simulink model "Controller"  (R2022b)
settings: Solver=FixedStepDiscrete  StartTime=0.0  StopTime=10.0  FixedStep=CONTROL_CONST.dt  RelTol=1e-3
values from neighbouring files (symbols this model uses):
  CONTROL_EXPORT = Simulink.Parameter(CONTROL_EXPORT_VALUE)    [controller_model_init.m]
  CONTROL_PARAM = Simulink.Parameter(CONTROL_PARAM_VALUE)    [controller_model_init.m]
undefined symbols (not defined in the file or in its folder): actuator_cmd, CONTROL_CONST, CONTROL_PARAM_VALUE, ControlMode, DiscIntNeverNeededParam, Discrete, Time, timestamp
libraries: simulink x10, FMT_Model_Lib x2, aerolibasang x1, ctrlSharedLib x1
(part 1 of 2)
settings Model: Creator=19114  LastModifiedBy=19114

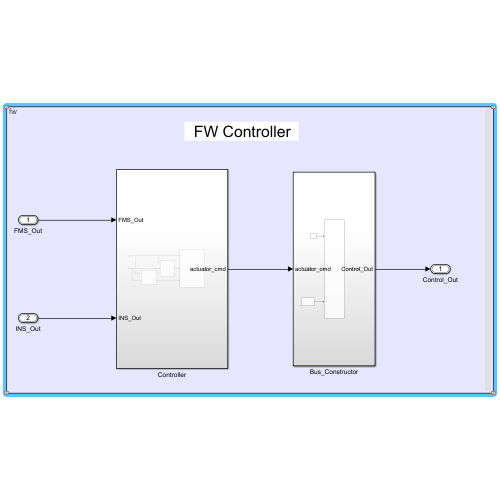
[thumbnail: Simulink's stored preview of the top-level diagram]
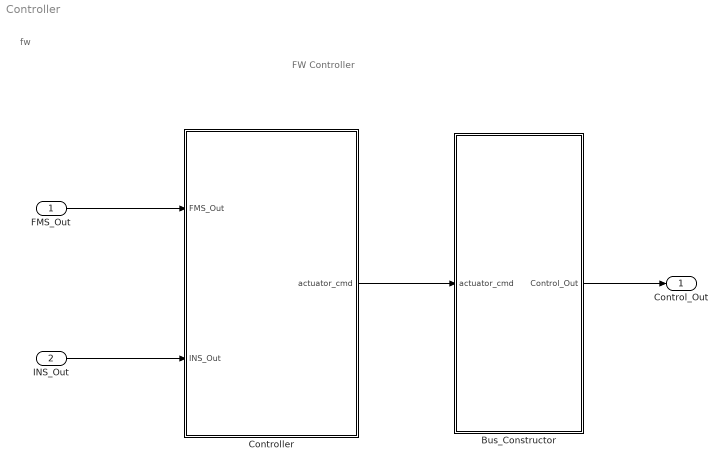
== system Controller ==
  note: FW Controller
  note: fw
  FMS_Out : Inport  OutDataTypeStr=Bus: FMS_Out_Bus
  INS_Out : Inport  Port=2  OutDataTypeStr=Bus: INS_Out_Bus
  Bus_Constructor : Subsystem
  Controller : Subsystem
  Control_Out : Outport  OutDataTypeStr=Bus: Control_Out_Bus  VectorParamsAs1DForOutWhenUnconnected=off
  wires:
  Bus_Constructor/1(Control_Out) -> Control_Out/1
  FMS_Out/1 -> Controller/1(FMS_Out)
  Controller/1(actuator_cmd) -> Bus_Constructor/1(actuator_cmd)
  INS_Out/1 -> Controller/2(INS_Out)

== system Controller/Bus_Constructor ==
  actuator_cmd : Inport
  Bus Assignment : BusAssignment  AssignedSignals=actuator_cmd,timestamp
  Constant : Constant  Value=0  OutDataTypeStr=Bus: Control_Out_Bus
  timestamp : Subsystem  mask{sample_time=CONTROL_EXPORT.period}
      mask prompts: sample_time "sample time (ms)"
  Control_Out : Outport  VectorParamsAs1DForOutWhenUnconnected=off
  wires:
  actuator_cmd/1 -> Bus Assignment/2
  timestamp/1(timestamp_ms) -> Bus Assignment/3
  Bus Assignment/1 -> Control_Out/1
  Constant/1 -> Bus Assignment/1

== system Controller/Controller ==
  FMS_Out : Inport
  INS_Out : Inport  Port=2
  Attitude_Control : Subsystem
  Control_Allocation : Subsystem  Variant=on  VariantActivationTime=code compile
  Lateral_Longitudinal_Control : Subsystem
  actuator_cmd : Outport  VectorParamsAs1DForOutWhenUnconnected=off
  wires:
  INS_Out/1 -> Attitude_Control/2(INS_Out), Lateral_Longitudinal_Control/2(INS_Out)
  Lateral_Longitudinal_Control/2(throttle_cmd) -> Control_Allocation/3(line_acc_cmd)
  Control_Allocation/1(actuator_cmd) -> actuator_cmd/1
  Attitude_Control/1(rate_dot_cmd) -> Control_Allocation/2(rate_dot_cmd)
  FMS_Out/1 -> Lateral_Longitudinal_Control/1(FMS_Out), Attitude_Control/1(FMS_Out), Control_Allocation/1(FMS_Out)
  Lateral_Longitudinal_Control/1(att_cmd) -> Attitude_Control/3(att_cmd)

== system Controller/Bus_Constructor/timestamp ==
  Constant : Constant  Value=sample_time
  Data Type Conversion : DataTypeConversion  OutDataTypeStr=uint32  SaturateOnIntegerOverflow=off  RndMeth=Floor
  Discrete-Time Integrator : DiscreteIntegrator  IntegratorMethod=Accumulation: Forward Euler  SampleTime=-1  ICPrevOutput=DiscIntNeverNeededParam  ICPrevScaledInput=DiscIntNeverNeededParam
  timestamp_ms : Outport  VectorParamsAs1DForOutWhenUnconnected=off
  wires:
  Discrete-Time Integrator/1 -> Data Type Conversion/1
  Constant/1 -> Discrete-Time Integrator/1
  Data Type Conversion/1 -> timestamp_ms/1

== system Controller/Controller/Attitude_Control ==
  FMS_Out : Inport
  INS_Out : Inport  Port=2
  att_cmd : Inport  Port=3
  Innerloop_Rate_Control : Subsystem
  Outloop_Angle_Control : Subsystem
  rate_dot_cmd : Outport  VectorParamsAs1DForOutWhenUnconnected=off
  wires:
  Outloop_Angle_Control/1(euler_rate_cmd) -> Innerloop_Rate_Control/1(euler_rate_cmd)
  INS_Out/1 -> Innerloop_Rate_Control/3(INS_Out), Outloop_Angle_Control/2(INS_Out)
  FMS_Out/1 -> Innerloop_Rate_Control/2(FMS_Out), Outloop_Angle_Control/3(FMS_Out)
  att_cmd/1 -> Outloop_Angle_Control/1(att_cmd)
  Innerloop_Rate_Control/1(rate_dot_cmd) -> rate_dot_cmd/1

== system Controller/Controller/Control_Allocation ==
  note: 1) Add Subsystem or Model blocks as valid variant choices.
      | 2) You cannot connect blocks at this level. At simulation, connectivity is automatically
      | determined, based on the active variant and port name matching.
  FMS_Out : Inport
  rate_dot_cmd : Inport  Port=2
  line_acc_cmd : Inport  Port=3
  Fixwing : Subsystem  TreatAsAtomicUnit=on  VariantControl=AIRFRAME==1
      mask Display: image('.\figures\fixwing.png');
  actuator_cmd : Outport  VectorParamsAs1DForOutWhenUnconnected=off

== system Controller/Controller/Lateral_Longitudinal_Control ==
  FMS_Out : Inport
  INS_Out : Inport  Port=2
  Airspeed_Filter : Subsystem
  Altitude_Control : Subsystem
  Lateral_Control : Subsystem
  Longitudinal_Control : Subsystem
  Mux : Mux  Inputs=2
  att_cmd : Outport  VectorParamsAs1DForOutWhenUnconnected=off
  throttle_cmd : Outport  Port=2  VectorParamsAs1DForOutWhenUnconnected=off
  wires:
  FMS_Out/1 -> Lateral_Control/1(FMS_Out), Longitudinal_Control/4(FMS_Out), Airspeed_Filter/1(FMS_Out), Altitude_Control/1(FMS_Out)
  Altitude_Control/1(alt_rate_sp) -> Longitudinal_Control/1(alt_rate_sp)
  INS_Out/1 -> Airspeed_Filter/2(INS), Altitude_Control/2(INS_Out)
  Longitudinal_Control/1(pitch_cmd) -> Mux/2  "pitch_cmd"
  Altitude_Control/2(alt_rate) -> Longitudinal_Control/2(alt_rate)
  Longitudinal_Control/2(throttle_cmd) -> throttle_cmd/1
  Airspeed_Filter/1(airspeed) -> Longitudinal_Control/3(airspeed)
  Lateral_Control/1(roll_cmd) -> Mux/1  "roll_cmd"
  Mux/1 -> att_cmd/1

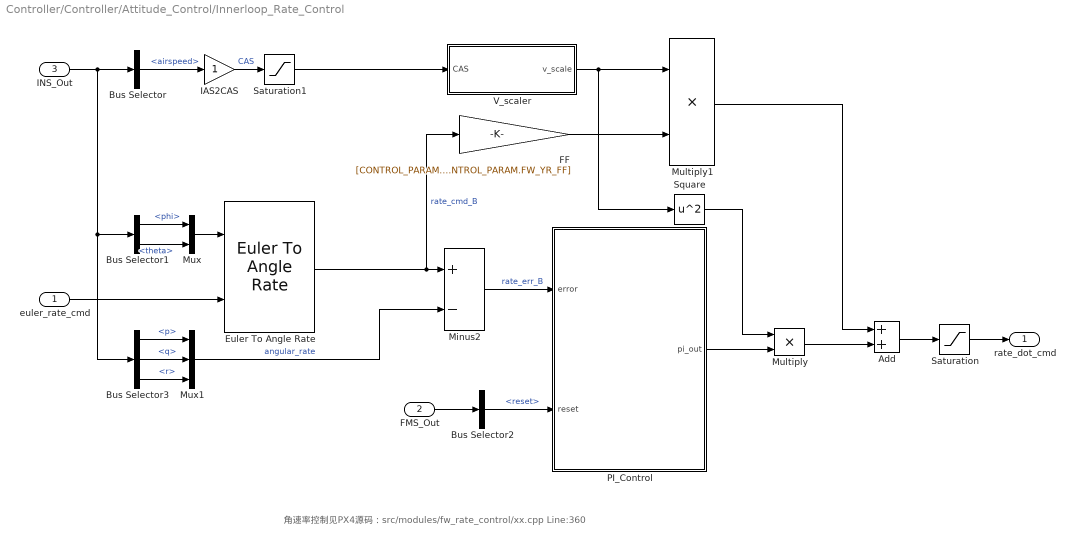
== system Controller/Controller/Attitude_Control/Innerloop_Rate_Control ==
  note: 角速率控制见PX4源码：src/modules/fw_rate_control/xx.cpp Line:360
  euler_rate_cmd : Inport
  FMS_Out : Inport  Port=2
  INS_Out : Inport  Port=3
  Add : Sum
  Bus Selector : BusSelector  OutputSignals=airspeed
  Bus Selector1 : BusSelector  OutputSignals=phi,theta
  Bus Selector2 : BusSelector  OutputSignals=reset
  Bus Selector3 : BusSelector  OutputSignals=p,q,r
  Euler To Angle Rate : FMT_Model_Lib/Math/Euler To Angle Rate
      settings: SourceProductName=FMT Toolbox
  FF : Gain  Gain=[CONTROL_PARAM.FW_RR_FF,CONTROL_PARAM.FW_PR_FF,CONTROL_PARAM.FW_YR_FF]
  IAS2CAS : Gain
  Minus2 : Sum  Inputs=+-
  Multiply : Product
  Multiply1 : Product
  Mux : Mux  Inputs=2
  Mux1 : Mux  Inputs=3
  PI_Control : Subsystem
  Saturation : Saturate  UpperLimit=1  LowerLimit=-1
  Saturation1 : Saturate  UpperLimit=inf  LowerLimit=0.5
  Square : Math  Operator=square
  V_scaler : Subsystem
  rate_dot_cmd : Outport  VectorParamsAs1DForOutWhenUnconnected=off
  wires:
  V_scaler/1(v_scale) -> Square/1, Multiply1/1
  FF/1 -> Multiply1/2
  Multiply1/1 -> Add/1
  Bus Selector/1 -> IAS2CAS/1  "<airspeed>"
  euler_rate_cmd/1 -> Euler To Angle Rate/2
  Euler To Angle Rate/1 -> FF/1, Minus2/1  "rate_cmd_B"
  Mux1/1 -> Minus2/2  "angular_rate"
  Multiply/1 -> Add/2
  Add/1 -> Saturation/1
  Minus2/1 -> PI_Control/1(error)  "rate_err_B"
  Bus Selector2/1 -> PI_Control/2(reset)  "<reset>"
  PI_Control/1(pi_out) -> Multiply/2
  INS_Out/1 -> Bus Selector/1, Bus Selector3/1, Bus Selector1/1
  Bus Selector1/1 -> Mux/1  "<phi>"
  Bus Selector1/2 -> Mux/2  "<theta>"
  Mux/1 -> Euler To Angle Rate/1
  FMS_Out/1 -> Bus Selector2/1
  Bus Selector3/1 -> Mux1/1  "<p>"
  Bus Selector3/2 -> Mux1/2  "<q>"
  Bus Selector3/3 -> Mux1/3  "<r>"
  Saturation1/1 -> V_scaler/1(CAS)
  IAS2CAS/1 -> Saturation1/1  "CAS"
  Square/1 -> Multiply/1
  Saturation/1 -> rate_dot_cmd/1

== system Controller/Controller/Attitude_Control/Outloop_Angle_Control ==
  att_cmd : Inport
  INS_Out : Inport  Port=2
  FMS_Out : Inport  Port=3
  Attitude_Controller : Subsystem
  Heading_Controller : Subsystem
  Mux : Mux  Inputs=2
  Reshape : Reshape  OutputDimensionality=Column vector (2-D)
  Signal_Select : Subsystem
  euler_rate_cmd : Outport  VectorParamsAs1DForOutWhenUnconnected=off
  wires:
  FMS_Out/1 -> Heading_Controller/3(FMS_Out), Signal_Select/2(FMS_Out)
  INS_Out/1 -> Heading_Controller/2(INS_Out), Attitude_Controller/2(INS_Out)
  att_cmd/1 -> Signal_Select/1(att_cmd_rad)
  Attitude_Controller/1(phi_theta_rate_cmd) -> Mux/1
  Heading_Controller/1(psi_rate_cmd) -> Mux/2
  Mux/1 -> Reshape/1
  Reshape/1 -> euler_rate_cmd/1
  Signal_Select/1(out) -> Heading_Controller/1(att_cmd), Attitude_Controller/1(att_cmd)

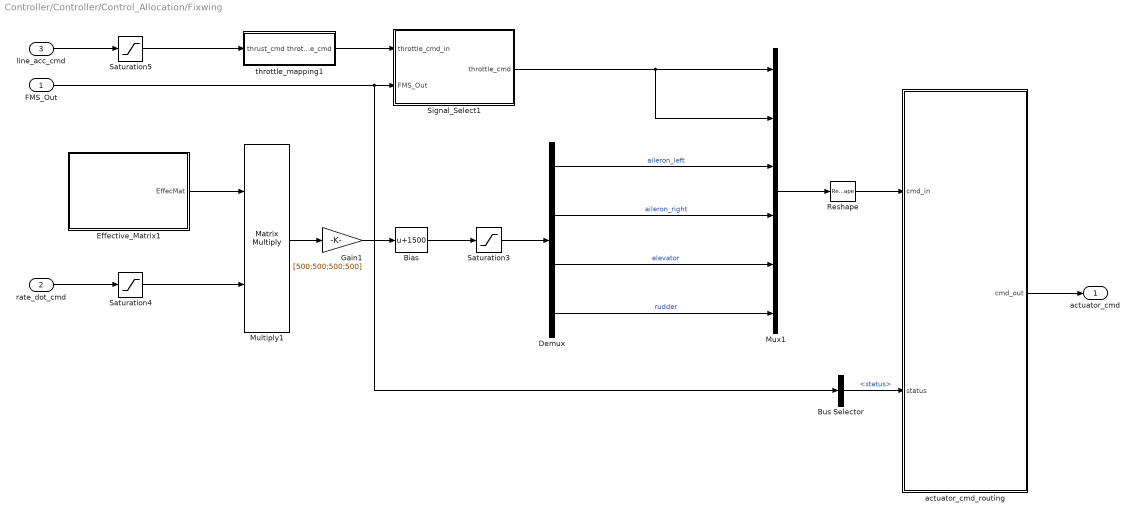
== system Controller/Controller/Control_Allocation/Fixwing ==
  FMS_Out : Inport
  rate_dot_cmd : Inport  Port=2
  line_acc_cmd : Inport  Port=3
  Bias : Bias  Bias=1500  SaturateOnIntegerOverflow=off
  Bus Selector : BusSelector  OutputSignals=status
  Demux : Demux
  Effective_Matrix1 : Subsystem
  Gain1 : Gain  Gain=[500;500;500;500]  OutDataTypeStr=Inherit: Same as input  ParamDataTypeStr=Inherit: Same as input
  Multiply1 : Product  Multiplication=Matrix(*)  OutDataTypeStr=Inherit: Same as first input
  Mux1 : Mux  Inputs=6
  Reshape : Reshape  OutputDimensionality=Column vector (2-D)  OutputDimensions=[16,1]
  Saturation3 : Saturate  UpperLimit=2000  LowerLimit=1000  OutDataTypeStr=uint16
  Saturation4 : Saturate  UpperLimit=1  LowerLimit=-1
  Saturation5 : Saturate  UpperLimit=1  LowerLimit=-1
  Signal_Select1 : Subsystem
  actuator_cmd_routing : Subsystem
  throttle_mapping1 : Subsystem
  actuator_cmd : Outport  VectorParamsAs1DForOutWhenUnconnected=off
  wires:
  rate_dot_cmd/1 -> Saturation4/1
  actuator_cmd_routing/1(cmd_out) -> actuator_cmd/1
  Bus Selector/1 -> actuator_cmd_routing/2(status)  "<status>"
  Demux/3 -> Mux1/5  "elevator"
  Demux/1 -> Mux1/3  "aileron_left"
  Saturation4/1 -> Multiply1/2
  Demux/4 -> Mux1/6  "rudder"
  Saturation3/1 -> Demux/1
  Demux/2 -> Mux1/4  "aileron_right"
  Multiply1/1 -> Gain1/1
  Effective_Matrix1/1(EffecMat) -> Multiply1/1
  Gain1/1 -> Bias/1
  Saturation5/1 -> throttle_mapping1/1(thrust_cmd)
  line_acc_cmd/1 -> Saturation5/1
  Signal_Select1/1(throttle_cmd) -> Mux1/2, Mux1/1
  Bias/1 -> Saturation3/1
  throttle_mapping1/1(throttle_cmd) -> Signal_Select1/1(throttle_cmd_in)
  Mux1/1 -> Reshape/1
  FMS_Out/1 -> Signal_Select1/2(FMS_Out), Bus Selector/1
  Reshape/1 -> actuator_cmd_routing/1(cmd_in)

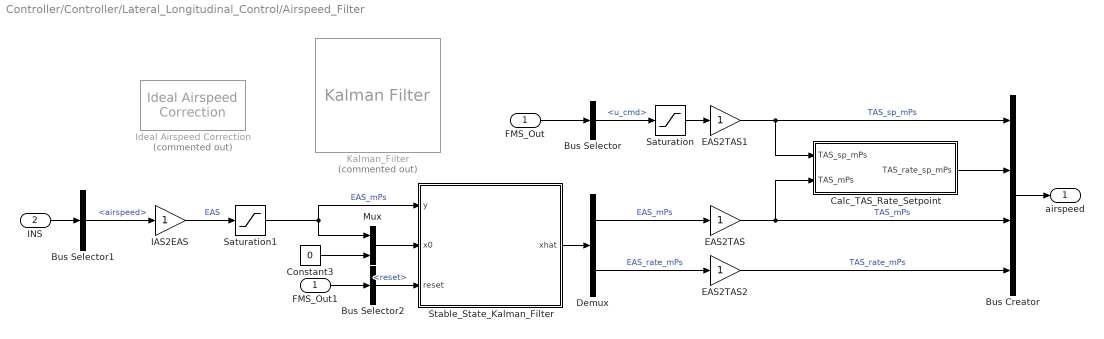
== system Controller/Controller/Lateral_Longitudinal_Control/Airspeed_Filter ==
  FMS_Out : Inport
  INS : Inport  Port=2
  Bus Creator : BusCreator  Inputs=4
  Bus Selector : BusSelector  OutputSignals=u_cmd
  Bus Selector1 : BusSelector  OutputSignals=airspeed
  Bus Selector2 : BusSelector  OutputSignals=reset
  Calc_TAS_Rate_Setpoint : Subsystem
  Constant3 : Constant  Value=0  OutDataTypeStr=single  LockScale=on
  Demux : Demux  Outputs=2
  EAS2TAS : Gain
  EAS2TAS1 : Gain
  EAS2TAS2 : Gain
  FMS_Out1 : InportShadow
  IAS2EAS : Gain
  Ideal Airspeed Correction : aerolibasang/Ideal Airspeed Correction  Commented=on  units=Metric (MKS)  vel_in=CAS  vel_out_tas=CAS  vel_out_eas=TAS  vel_out_cas=TAS  method=Table Lookup  SubOnly=on  action=None
  Kalman_Filter : ctrlSharedLib/Kalman Filter  Commented=on  TimeDomain=Discrete-Time  UseCurrentEstimator=off  ModelSource=Individual A, B, C, D matrices  ModelSourceVariable=ss(0.95,1,1,0,1)  A=[1 CONTROL_CONST.dt;0 1]  B=1  C=[1 0]  D=0  NumberOfStates=1  NumberOfInputs=1  NumberOfOutputs=1  InitialEstimateSource=Input port  X0=0  P0=10  UseK=off  UseGH=off  NumberOfProcessNoiseInputs=1  G=1  TimeInvariantG=on  H=[1 0]  TimeInvariantH=on  Q=CONTROL_PARAM.FW_T_SPD_PRC_STD  TimeInvariantQ=on  R=CONTROL_PARAM.FW_T_SPD_STD  TimeInvariantR=on  N=0  TimeInvariantN=on  AddInputPort=off  AddEnablePort=off  ExternalReset=Level  OutputEstimatedY=off  OutputP=off  Ts=CONTROL_CONST.dt
  Mux : Mux  Inputs=2
  Saturation : Saturate  UpperLimit=CONTROL_PARAM.FW_AIRSPD_MAX  LowerLimit=CONTROL_PARAM.FW_AIRSPD_MIN
  Saturation1 : Saturate  UpperLimit=inf  LowerLimit=0
  Stable_State_Kalman_Filter : Subsystem  mask{r1=0.2, r2=0.2, q=0.2, dt=CONTROL_CONST.dt}
      mask prompts: r1 "airspeed measurement standard deviation in [m/s]"; r2 "airspeed rate measurement standard deviation in [m/s²]"; q "standard deviation on the airspeed rate deviation in the model in [m/s²]"; dt "SampleTime"
      mask DialogControl DescGroupVar Prompt: Airspeed Filter
      mask DialogControl DescTextVar Prompt: Filter airspeed and rate using a constant airspeed rate model in a steady state Kalman Filter.
      mask DialogControl ParameterGroupVar Prompt: 参数
      mask Display:
      | port_label('input', 1, 'y');
      | port_label('input', 2, 'x0');
      | port_label('input', 3, 'reset');
      | port_label('output', 1, 'xhat');
      | disp('Airspeed Filter');
  airspeed : Outport
  wires:
  Bus Selector1/1 -> IAS2EAS/1  "<airspeed>"
  INS/1 -> Bus Selector1/1
  IAS2EAS/1 -> Saturation1/1  "EAS"
  Bus Creator/1 -> airspeed/1
  Saturation1/1 -> Stable_State_Kalman_Filter/1(y), Mux/1  "EAS_mPs"
  Constant3/1 -> Mux/2
  Stable_State_Kalman_Filter/1(xhat) -> Demux/1
  Demux/1 -> EAS2TAS/1  "EAS_mPs"
  Demux/2 -> EAS2TAS2/1  "EAS_rate_mPs"
  EAS2TAS/1 -> Calc_TAS_Rate_Setpoint/2(TAS_mPs), Bus Creator/3  "TAS_mPs"
  Mux/1 -> Stable_State_Kalman_Filter/2(x0)
  FMS_Out/1 -> Bus Selector/1
  EAS2TAS1/1 -> Calc_TAS_Rate_Setpoint/1(TAS_sp_mPs), Bus Creator/1  "TAS_sp_mPs"
  Bus Selector/1 -> Saturation/1  "<u_cmd>"
  Saturation/1 -> EAS2TAS1/1
  EAS2TAS2/1 -> Bus Creator/4  "TAS_rate_mPs"
  Bus Selector2/1 -> Stable_State_Kalman_Filter/3(reset)  "<reset>"
  FMS_Out1/1 -> Bus Selector2/1
  Calc_TAS_Rate_Setpoint/1(TAS_rate_sp_mPs) -> Bus Creator/2

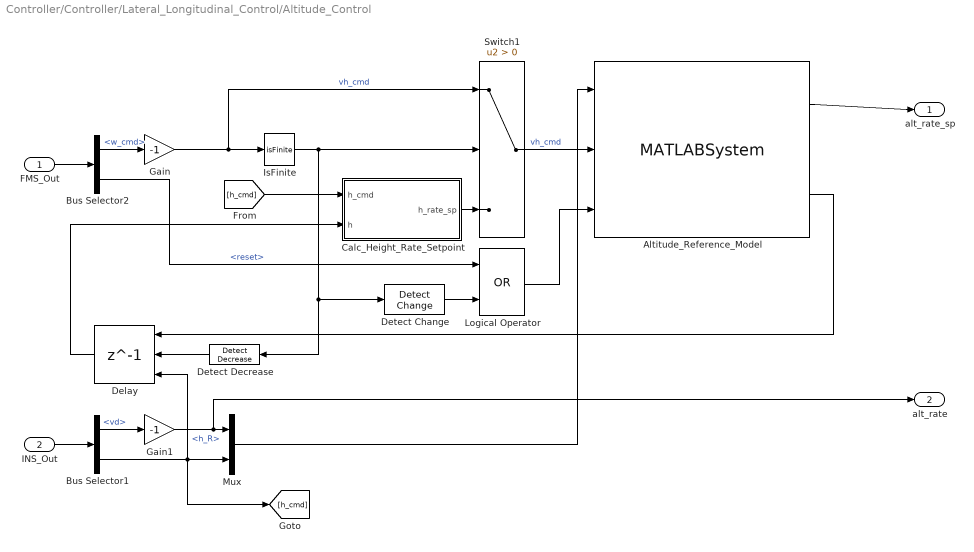
== system Controller/Controller/Lateral_Longitudinal_Control/Altitude_Control ==
  FMS_Out : Inport
  INS_Out : Inport  Port=2
  Altitude_Reference_Model : MATLABSystem  System=VelocitySmoothing  max_jerk=single(1000)  max_accel=CONTROL_PARAM.FW_T_VERT_ACC  max_climb_rate=CONTROL_PARAM.FW_T_CLMB_MAX  max_sink_rate=CONTROL_PARAM.FW_T_SINK_MAX  SampleTime=CONTROL_CONST.dt  SimulateUsing=Code generation
      mask Type: VelocitySmoothing
      mask Display:
      | disp(['Velocity' char(10) 'Smoothing']);
      | port_label('input',1,'v0x0');
      | port_label('input',2,'vel_sp');
      | port_label('input',3,'reset');
      | port_label('output',1,'vel');
      | port_label('output',2,'pos');
  Bus Selector1 : BusSelector  OutputSignals=vd,h_R
  Bus Selector2 : BusSelector  OutputSignals=w_cmd,reset
  Calc_Height_Rate_Setpoint : Subsystem
  Delay : Delay  DelayLength=1  InitialConditionSource=Input port  ExternalReset=Level
      settings: InputPortMap=u0,r5,p4
  Detect Change : simulink/Logic and Bit Operations/Detect Change  vinit=0  OutDataTypeStr=boolean
  Detect Decrease : simulink/Logic and Bit Operations/Detect Decrease  vinit=0.0  OutDataTypeStr=boolean
  Gain : Gain  Gain=-1
  Gain1 : Gain  Gain=-1
  IsFinite : RelationalOperator  Operator=isFinite  OutDataTypeStr=boolean  RndMeth=Simplest  InputSameDT=off
  Logical Operator : Logic  Operator=OR  AllPortsSameDT=off  OutDataTypeStr=boolean
  Mux : Mux  Inputs=2
  Switch1 : Switch  Criteria=u2 > Threshold  SaturateOnIntegerOverflow=off  InputSameDT=off
  alt_rate_sp : Outport
  alt_rate : Outport  Port=2
  wires:
  FMS_Out/1 -> Bus Selector2/1
  INS_Out/1 -> Bus Selector1/1
  Bus Selector1/2 -> Mux/2, [h_cmd], Delay/3  "<h_R>"
  Bus Selector2/1 -> Gain/1  "<w_cmd>"
  Gain/1 -> IsFinite/1, Switch1/1  "vh_cmd"
  IsFinite/1 -> Detect Decrease/1, Detect Change/1, Switch1/2
  Bus Selector1/1 -> Gain1/1  "<vd>"
  Gain1/1 -> alt_rate/1, Mux/1
  Detect Change/1 -> Logical Operator/2
  Mux/1 -> Altitude_Reference_Model/1
  Switch1/1 -> Altitude_Reference_Model/2  "vh_cmd"
  Logical Operator/1 -> Altitude_Reference_Model/3
  Altitude_Reference_Model/2 -> Delay/1
  [h_cmd] -> Calc_Height_Rate_Setpoint/1(h_cmd)
  Delay/1 -> Calc_Height_Rate_Setpoint/2(h)
  Calc_Height_Rate_Setpoint/1(h_rate_sp) -> Switch1/3
  Detect Decrease/1 -> Delay/2
  Altitude_Reference_Model/1 -> alt_rate_sp/1
  Bus Selector2/2 -> Logical Operator/1  "<reset>"

== system Controller/Controller/Lateral_Longitudinal_Control/Lateral_Control ==
  FMS_Out : Inport
  Atan : Trigonometry  Operator=atan
  Bus Selector : BusSelector  OutputSignals=ay_cmd
  Constant : Constant  Value=CONTROL_CONST.g
  Product : Product  Inputs=/*
  Saturation : Saturate  UpperLimit=CONTROL_PARAM.FW_R_LIM  LowerLimit=-CONTROL_PARAM.FW_R_LIM
  roll_cmd : Outport
  wires:
  FMS_Out/1 -> Bus Selector/1
  Constant/1 -> Product/1
  Bus Selector/1 -> Product/2  "<ay_cmd>"
  Product/1 -> Atan/1
  Atan/1 -> Saturation/1
  Saturation/1 -> roll_cmd/1

== system Controller/Controller/Lateral_Longitudinal_Control/Longitudinal_Control ==
  alt_rate_sp : Inport
  alt_rate : Inport  Port=2
  airspeed : Inport  Port=3
  FMS_Out : Inport  Port=4
  Calc_Specific_Energy_Rates : Subsystem
  Pitch_Control : Subsystem
  Throttle_Control : Subsystem
  pitch_cmd : Outport
  throttle_cmd : Outport  Port=2
  wires:
  alt_rate_sp/1 -> Calc_Specific_Energy_Rates/1(alt_rate_sp)
  airspeed/1 -> Pitch_Control/3(airspeed), Calc_Specific_Energy_Rates/3(airspeed)
  alt_rate/1 -> Calc_Specific_Energy_Rates/2(alt_rate)
  Throttle_Control/1(throttle_cmd) -> throttle_cmd/1
  Pitch_Control/1(pitch_cmd) -> pitch_cmd/1
  FMS_Out/1 -> Pitch_Control/2(FMS_Out), Throttle_Control/2(FMS_Out)
  Calc_Specific_Energy_Rates/1(ser) -> Throttle_Control/1(ser), Pitch_Control/1(ser)

== system Controller/Controller/Attitude_Control/Innerloop_Rate_Control/PI_Control ==
  error : Inport
  reset : Inport  Port=2
  Add1 : Sum
  I_Control : Subsystem  mask{p_ki=CONTROL_PARAM.ROLL_RATE_I, q_ki=CONTROL_PARAM.PITCH_RATE_I, r_ki=CONTROL_PARAM.YAW_RATE_I, max_i=CONTROL_PARAM.RATE_I_MAX, min_i=CONTROL_PARAM.RATE_I_MIN}
  P_Control : Subsystem  mask{p_kp=CONTROL_PARAM.ROLL_RATE_P, q_kp=CONTROL_PARAM.PITCH_RATE_P, r_kp=CONTROL_PARAM.YAW_RATE_P}
  pi_out : Outport  VectorParamsAs1DForOutWhenUnconnected=off
  wires:
  Add1/1 -> pi_out/1
  I_Control/1(i_out) -> Add1/2  "i_out"
  error/1 -> P_Control/1(err), I_Control/1(err)
  P_Control/1(p_out) -> Add1/1
  reset/1 -> I_Control/2(reset)

== system Controller/Controller/Attitude_Control/Innerloop_Rate_Control/V_scaler ==
  CAS : Inport
  CAS_constrained : Saturate  UpperLimit=CONTROL_PARAM.FW_AIRSPD_MAX  LowerLimit=CONTROL_PARAM.FW_AIRSPD_STALL
  Constant1 : Constant  Value=CONTROL_PARAM.FW_ARSP_SCALE_EN
  Constant2 : Constant  OutDataTypeStr=single
  Divide : Product  Inputs=/*
  Switch1 : Switch  Criteria=u2 > Threshold  SaturateOnIntegerOverflow=off  InputSameDT=off
  Trim_CAS : Constant  Value=CONTROL_PARAM.FW_AIRSPD_TRIM
  v_scale : Outport
  wires:
  CAS_constrained/1 -> Divide/1
  Divide/1 -> Switch1/1
  Constant1/1 -> Switch1/2
  Switch1/1 -> v_scale/1
  Trim_CAS/1 -> Divide/2
  Constant2/1 -> Switch1/3
  CAS/1 -> CAS_constrained/1

== system Controller/Controller/Attitude_Control/Outloop_Angle_Control/Attitude_Controller ==
  att_cmd : Inport
  INS_Out : Inport  Port=2
  Error : Subsystem
  P_Controller : Subsystem
  phi_theta_rate_cmd : Outport  VectorParamsAs1DForOutWhenUnconnected=off
  wires:
  INS_Out/1 -> Error/2(INS_Out)
  P_Controller/1(u) -> phi_theta_rate_cmd/1
  att_cmd/1 -> Error/1(att_cmd)
  Error/1(euler_err_rad) -> P_Controller/1(error)

== system Controller/Controller/Attitude_Control/Outloop_Angle_Control/Heading_Controller ==
  att_cmd : Inport
  INS_Out : Inport  Port=2
  FMS_Out : Inport  Port=3
  Bus Selector2 : BusSelector  OutputSignals=psi_rate_cmd
  Selector : Selector  InputPortWidth=2  IndexOptions=Index vector (dialog)  Indices=[1]  OutputSizes=1
  Sum : Sum  Inputs=++|
  Turning_Coordination : Subsystem
  psi_rate_cmd : Outport  VectorParamsAs1DForOutWhenUnconnected=off
  wires:
  Turning_Coordination/1(psi_rate_sp) -> Sum/2
  Sum/1 -> psi_rate_cmd/1
  FMS_Out/1 -> Bus Selector2/1
  Bus Selector2/1 -> Sum/1  "<psi_rate_cmd>"
  INS_Out/1 -> Turning_Coordination/2(INS_Out)
  att_cmd/1 -> Selector/1
  Selector/1 -> Turning_Coordination/1(phi_sp)

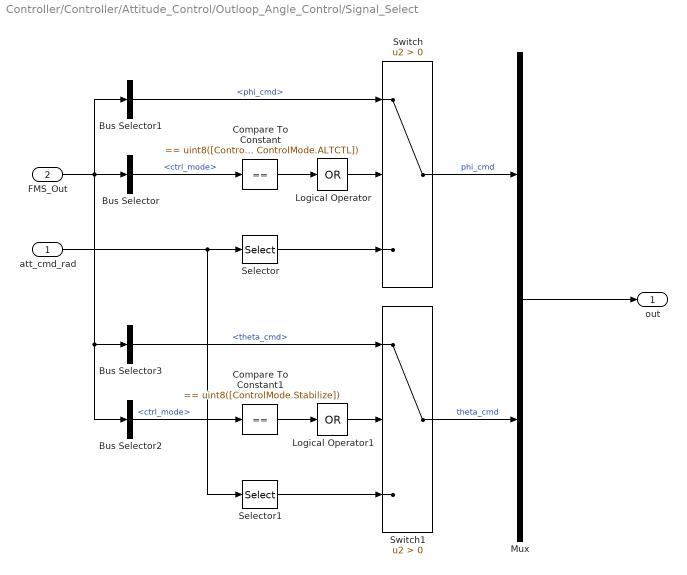
== system Controller/Controller/Attitude_Control/Outloop_Angle_Control/Signal_Select ==
  att_cmd_rad : Inport
  FMS_Out : Inport  Port=2
  Bus Selector : BusSelector  OutputSignals=ctrl_mode
  Bus Selector1 : BusSelector  OutputSignals=phi_cmd
  Bus Selector2 : BusSelector  OutputSignals=ctrl_mode
  Bus Selector3 : BusSelector  OutputSignals=theta_cmd
  Compare To Constant : simulink/Logic and Bit Operations/Compare To Constant  relop===  const=uint8([ControlMode.Stabilize, ControlMode.ALTCTL])  OutDataTypeStr=boolean
  Compare To Constant1 : simulink/Logic and Bit Operations/Compare To Constant  relop===  const=uint8([ControlMode.Stabilize])  OutDataTypeStr=boolean
  Logical Operator : Logic  Operator=OR  Inputs=1  AllPortsSameDT=off  OutDataTypeStr=boolean
  Logical Operator1 : Logic  Operator=OR  Inputs=1  AllPortsSameDT=off  OutDataTypeStr=boolean
  Mux : Mux  Inputs=2
  Selector : Selector  InputPortWidth=2  IndexOptions=Index vector (dialog)  Indices=1  OutputSizes=1
  Selector1 : Selector  InputPortWidth=2  IndexOptions=Index vector (dialog)  Indices=2  OutputSizes=1
  Switch : Switch  Criteria=u2 > Threshold  SaturateOnIntegerOverflow=off  InputSameDT=off
  Switch1 : Switch  Criteria=u2 > Threshold  SaturateOnIntegerOverflow=off  InputSameDT=off
  out : Outport  VectorParamsAs1DForOutWhenUnconnected=off
  wires:
  Compare To Constant/1 -> Logical Operator/1
  att_cmd_rad/1 -> Selector/1, Selector1/1
  Bus Selector/1 -> Compare To Constant/1  "<ctrl_mode>"
  FMS_Out/1 -> Bus Selector2/1, Bus Selector3/1, Bus Selector1/1, Bus Selector/1
  Bus Selector1/1 -> Switch/1  "<phi_cmd>"
  Logical Operator/1 -> Switch/2
  Selector/1 -> Switch/3
  Logical Operator1/1 -> Switch1/2
  Compare To Constant1/1 -> Logical Operator1/1
  Bus Selector2/1 -> Compare To Constant1/1  "<ctrl_mode>"
  Bus Selector3/1 -> Switch1/1  "<theta_cmd>"
  Selector1/1 -> Switch1/3
  Switch/1 -> Mux/1  "phi_cmd"
  Switch1/1 -> Mux/2  "theta_cmd"
  Mux/1 -> out/1

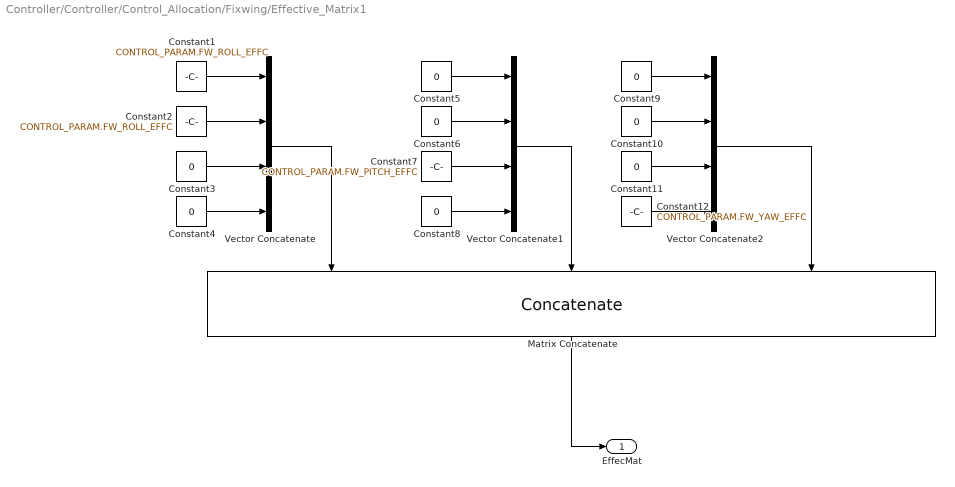
== system Controller/Controller/Control_Allocation/Fixwing/Effective_Matrix1 ==
  Constant1 : Constant  Value=CONTROL_PARAM.FW_ROLL_EFFC  OutDataTypeStr=single
  Constant{3..6,8..11} (8 alike) : Constant  Value=0  OutDataTypeStr=single
  Constant12 : Constant  Value=CONTROL_PARAM.FW_YAW_EFFC  OutDataTypeStr=single
  Constant2 : Constant  Value=CONTROL_PARAM.FW_ROLL_EFFC  OutDataTypeStr=single
  Constant7 : Constant  Value=CONTROL_PARAM.FW_PITCH_EFFC  OutDataTypeStr=single
  Matrix Concatenate : Concatenate  NumInputs=3  Mode=Multidimensional array  ConcatenateDimension=2
  Vector Concatenate : Concatenate  NumInputs=4
  Vector Concatenate1 : Concatenate  NumInputs=4
  Vector Concatenate2 : Concatenate  NumInputs=4
  EffecMat : Outport  VectorParamsAs1DForOutWhenUnconnected=off
  wires:
  Constant7/1 -> Vector Concatenate1/3
  Constant8/1 -> Vector Concatenate1/4
  Constant9/1 -> Vector Concatenate2/1
  Constant12/1 -> Vector Concatenate2/4
  Constant3/1 -> Vector Concatenate/3
  Vector Concatenate/1 -> Matrix Concatenate/1
  Matrix Concatenate/1 -> EffecMat/1
  Constant2/1 -> Vector Concatenate/2
  Constant11/1 -> Vector Concatenate2/3
  Constant10/1 -> Vector Concatenate2/2
  Constant1/1 -> Vector Concatenate/1
  Vector Concatenate2/1 -> Matrix Concatenate/3
  Constant4/1 -> Vector Concatenate/4
  Vector Concatenate1/1 -> Matrix Concatenate/2
  Constant5/1 -> Vector Concatenate1/1
  Constant6/1 -> Vector Concatenate1/2

== system Controller/Controller/Control_Allocation/Fixwing/Signal_Select1 ==
  throttle_cmd_in : Inport
  FMS_Out : Inport  Port=2
  Bus Selector1 : BusSelector  OutputSignals=throttle_cmd,ctrl_mode
  Compare To Constant : simulink/Logic and Bit Operations/Compare To Constant  relop===  const=uint8([ControlMode.Manual, ControlMode.Acro, ControlMode.Stabilize])  OutDataTypeStr=boolean
  Logical Operator : Logic  Operator=OR  Inputs=1  AllPortsSameDT=off  OutDataTypeStr=boolean
  Switch : Switch  Criteria=u2 > Threshold  SaturateOnIntegerOverflow=off  InputSameDT=off
  throttle_cmd : Outport  VectorParamsAs1DForOutWhenUnconnected=off
  wires:
  Logical Operator/1 -> Switch/2
  throttle_cmd_in/1 -> Switch/3
  Switch/1 -> throttle_cmd/1  "throttle_cmd"
  Bus Selector1/2 -> Compare To Constant/1  "<ctrl_mode>"
  Bus Selector1/1 -> Switch/1  "<throttle_cmd>"
  FMS_Out/1 -> Bus Selector1/1
  Compare To Constant/1 -> Logical Operator/1

== system Controller/Controller/Control_Allocation/Fixwing/actuator_cmd_routing ==
  cmd_in : Inport
  status : Inport  Port=2
  Constant : Constant  Value=zeros(10,1)  VectorParams1D=off  OutDataTypeStr=uint16
  Disarm : Constant  Value=[1000 1000 1500 1500 1500 1500]'  VectorParams1D=off  OutDataTypeStr=uint16
  Multiport Switch : MultiPortSwitch  DataPortForDefault=Additional data port  DiagnosticForDefault=None  SaturateOnIntegerOverflow=off  InputSameDT=off
  Mux1 : Mux  Inputs=2
  Reshape : Reshape  OutputDimensionality=Customize  OutputDimensions=[16,1]
  Standby : Constant  Value=[1050 1050 1500 1500 1500 1500]'  VectorParams1D=off  OutDataTypeStr=uint16
  cmd_out : Outport  VectorParamsAs1DForOutWhenUnconnected=off
  wires:
  Disarm/1 -> Multiport Switch/5, Multiport Switch/2
  Reshape/1 -> cmd_out/1
  Constant/1 -> Mux1/2
  Standby/1 -> Multiport Switch/3
  Mux1/1 -> Reshape/1
  status/1 -> Multiport Switch/1
  Multiport Switch/1 -> Mux1/1
  cmd_in/1 -> Multiport Switch/4

== system Controller/Controller/Control_Allocation/Fixwing/throttle_mapping1 ==
  thrust_cmd : Inport
  Constant1 : Constant  Value=1000  OutDataTypeStr=uint32
  Data Type Conversion : DataTypeConversion  OutDataTypeStr=uint16  SaturateOnIntegerOverflow=off  RndMeth=Floor
  Gain1 : Gain  Gain=1000  OutDataTypeStr=uint32
  Saturation : Saturate  UpperLimit=1  LowerLimit=0
  Sum1 : Sum  Inputs=|++
  throttle_cmd : Outport  VectorParamsAs1DForOutWhenUnconnected=off
  wires:
  Sum1/1 -> Data Type Conversion/1
  thrust_cmd/1 -> Saturation/1
  Data Type Conversion/1 -> throttle_cmd/1
  Constant1/1 -> Sum1/2
  Gain1/1 -> Sum1/1
  Saturation/1 -> Gain1/1

== system Controller/Controller/Lateral_Longitudinal_Control/Airspeed_Filter/Calc_TAS_Rate_Setpoint ==
  TAS_sp_mPs : Inport
  TAS_mPs : Inport  Port=2
  Constant : Constant  Value=CONTROL_CONST.g*CONTROL_PARAM.FW_T_CLMB_MAX*0.5  OutDataTypeStr=single
  Constant1 : Constant  Value=CONTROL_CONST.g*CONTROL_PARAM.FW_T_SINK_MIN*0.5  OutDataTypeStr=single
  Product : Product  Inputs=*/
  Product1 : Product  Inputs=/*
  Saturation Dynamic : simulink/Discontinuities/Saturation Dynamic  OutMin=[]  OutMax=[]  OutDataTypeStr=Inherit: Same as second input  OutDataType=fixdt(1, 16)  OutScaling=2^-10  DoSatur=off
  Sum : Sum  Inputs=|+-
  airspeed_error_gain : Gain  Gain=1/CONTROL_PARAM_VALUE.FW_T_TAS_TC
  TAS_rate_sp_mPs : Outport
  wires:
  Saturation Dynamic/1 -> TAS_rate_sp_mPs/1  "TAS_rate_sp_mPs"
  Sum/1 -> airspeed_error_gain/1
  TAS_sp_mPs/1 -> Sum/1
  TAS_mPs/1 -> Product/2, Product1/1, Sum/2
  airspeed_error_gain/1 -> Saturation Dynamic/2
  Constant/1 -> Product/1
  Product/1 -> Saturation Dynamic/1
  Product1/1 -> Saturation Dynamic/3
  Constant1/1 -> Product1/2

== system Controller/Controller/Lateral_Longitudinal_Control/Airspeed_Filter/Stable_State_Kalman_Filter ==
  y : Inport
  x0 : Inport  Port=2
  reset : Inport  Port=3
  A : Constant  Value=[1 dt;0 1]  OutDataTypeStr=single
  Add : Sum
  Add1 : Sum  Inputs=+-
  "Cal_K " : Subsystem
  Delay : Delay  DelayLength=1  InitialConditionSource=Input port  ExternalReset=Level  SampleTime=dt
      settings: InputPortMap=u0,r5,p4
  Matrix Multiply : Product  Multiplication=Matrix(*)
  Matrix Multiply1 : Product  Multiplication=Matrix(*)
  xhat : Outport
  wires:
  A/1 -> Matrix Multiply/1
  y/1 -> Add1/1
  Matrix Multiply/1 -> Add1/2, Add/2
  Add/1 -> xhat/1, Delay/1
  "Cal_K "/1(k_gain) -> Matrix Multiply1/1
  Delay/1 -> Matrix Multiply/2
  Add1/1 -> Matrix Multiply1/2
  Matrix Multiply1/1 -> Add/1
  x0/1 -> Delay/3
  reset/1 -> Delay/2

== system Controller/Controller/Lateral_Longitudinal_Control/Altitude_Control/Calc_Height_Rate_Setpoint ==
  note: Saturation
  h_cmd : Inport
  h : Inport  Port=2
  Abs : Abs  SaturateOnIntegerOverflow=off
  Constant2 : Constant  Value=1000  OutDataTypeStr=single
  Constant3 : Constant  Value=CONTROL_PARAM.FW_T_VERT_ACC  OutDataTypeStr=single
  Constant4 : Constant  Value=0  OutDataTypeStr=single
  Product : Product
  Saturation : Saturate  UpperLimit=min(CONTROL_PARAM.FW_T_CLMB_R_SP, CONTROL_PARAM.FW_T_CLMB_MAX)  LowerLimit=-min(CONTROL_PARAM.FW_T_SINK_R_SP, CONTROL_PARAM.FW_T_SINK_MAX)
  Sum : Sum  Inputs=|+-  OutDataTypeStr=Inherit: Same as first input
  computeMaxSpeedFromDistance : MATLAB Function  TreatAsAtomicUnit=on
  signNoZero : MATLAB Function  TreatAsAtomicUnit=on
  h_rate_sp : Outport  OutDataTypeStr=single
  wires:
  computeMaxSpeedFromDistance/1(max_speed) -> Product/1
  Constant3/1 -> computeMaxSpeedFromDistance/2(accel)
  h/1 -> Sum/2
  Sum/1 -> Abs/1, signNoZero/1(u)  "delta_m"
  Abs/1 -> computeMaxSpeedFromDistance/3(braking_distance)
  Constant2/1 -> computeMaxSpeedFromDistance/1(jerk)
  Constant4/1 -> computeMaxSpeedFromDistance/4(final_speed)
  signNoZero/1(y) -> Product/2
  h_cmd/1 -> Sum/1
  Product/1 -> Saturation/1
  Saturation/1 -> h_rate_sp/1

== system Controller/Controller/Lateral_Longitudinal_Control/Longitudinal_Control/Calc_Specific_Energy_Rates ==
  alt_rate_sp : Inport
  alt_rate : Inport  Port=2
  airspeed : Inport  Port=3
  Bus Creator : BusCreator  Inputs=4
  Bus Selector : BusSelector  OutputSignals=TAS_mPs,TAS_rate_sp_mPs,TAS_rate_mPs
  Constant : Constant  Value=CONTROL_CONST.g
  Product{1..4} (4 alike) : Product
  ser : Outport
  wires:
  Product4/1 -> Bus Creator/1  "spe_rate_sp"
  airspeed/1 -> Bus Selector/1
  Bus Selector/1 -> Product3/2, Product1/1  "<TAS_mPs>"
  Bus Selector/2 -> Product1/2  "<TAS_rate_sp_mPs>"
  Product1/1 -> Bus Creator/3  "ske_rate_sp"
  Bus Selector/3 -> Product3/1  "<TAS_rate_mPs>"
  Product2/1 -> Bus Creator/2  "spe_rate"
  Product3/1 -> Bus Creator/4  "ske_rate"
  Bus Creator/1 -> ser/1
  Constant/1 -> Product4/2, Product2/1
  alt_rate/1 -> Product2/2
  alt_rate_sp/1 -> Product4/1

== system Controller/Controller/Lateral_Longitudinal_Control/Longitudinal_Control/Pitch_Control ==
  ser : Inport
  FMS_Out : Inport  Port=2
  airspeed : Inport  Port=3
  Add : Sum
  Bus Selector : BusSelector  OutputSignals=TAS_mPs
  Bus Selector1 : BusSelector  OutputSignals=reset
  Calc_Seb_Rate : Subsystem
  Delay : Delay  DelayLength=1
  FF & Damp : Subsystem
  I : Subsystem
  Limit_Select : Subsystem
  Pitch_Saturation : Subsystem
  pitch_cmd : Outport
  wires:
  ser/1 -> Calc_Seb_Rate/1(ser)
  Calc_Seb_Rate/1(seb_rate_err) -> FF & Damp/1(seb_rate_err), I/1(err)
  I/1(i_out) -> Add/2
  Delay/1 -> Pitch_Saturation/4(cmd_last), I/4(cmd_last)
  Calc_Seb_Rate/2(seb_rate_sp) -> FF & Damp/2(seb_rate_sp)
  FF & Damp/1(ff_d_out) -> Add/1
  Pitch_Saturation/1(pitch_cmd) -> pitch_cmd/1, Delay/1
  airspeed/1 -> Bus Selector/1
  Add/1 -> Pitch_Saturation/2(ctrl_out)
  Bus Selector/1 -> Pitch_Saturation/1(tas)  "<TAS_mPs>"
  Limit_Select/1(maxmin) -> Pitch_Saturation/3(maxmin), I/2(maxmin)
  FMS_Out/1 -> Bus Selector1/1, Limit_Select/1(FMS_Out)
  Bus Selector1/1 -> I/3(reset)  "<reset>"

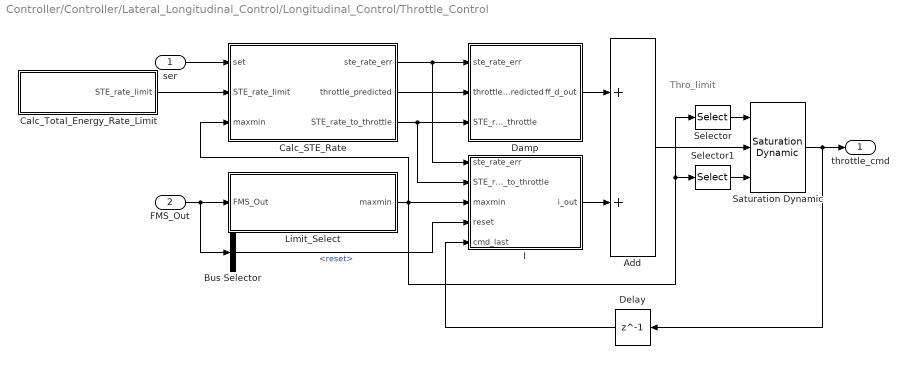
== system Controller/Controller/Lateral_Longitudinal_Control/Longitudinal_Control/Throttle_Control ==
  note: Thro_limit
  ser : Inport
  FMS_Out : Inport  Port=2
  Add : Sum
  Bus Selector : BusSelector  OutputSignals=reset
  Calc_STE_Rate : Subsystem
  Calc_Total_Energy_Rate_Limit : Subsystem
  Damp : Subsystem
  Delay : Delay  DelayLength=1
  I : Subsystem
  Limit_Select : Subsystem
  Saturation Dynamic : simulink/Discontinuities/Saturation Dynamic  OutMin=[]  OutMax=[]  OutDataTypeStr=Inherit: Same as second input  OutDataType=fixdt(1, 16)  OutScaling=2^-10  DoSatur=off
  Selector : Selector  InputPortWidth=2  IndexOptions=Index vector (dialog)  Indices=[1]  OutputSizes=1
  Selector1 : Selector  InputPortWidth=2  IndexOptions=Index vector (dialog)  Indices=[2]  OutputSizes=1
  throttle_cmd : Outport
  wires:
  Calc_Total_Energy_Rate_Limit/1(STE_rate_limit) -> Calc_STE_Rate/2(STE_rate_limit)
  ser/1 -> Calc_STE_Rate/1(set)
  I/1(i_out) -> Add/2
  Delay/1 -> I/5(cmd_last)
  Add/1 -> Saturation Dynamic/2
  Calc_STE_Rate/2(throttle_predicted) -> Damp/2(throttle_predicted)
  Saturation Dynamic/1 -> Delay/1, throttle_cmd/1
  Calc_STE_Rate/1(ste_rate_err) -> I/1(ste_rate_err), Damp/1(ste_rate_err)
  Damp/1(ff_d_out) -> Add/1
  Limit_Select/1(maxmin) -> I/3(maxmin), Selector1/1, Selector/1, Calc_STE_Rate/3(maxmin)
  Calc_STE_Rate/3(STE_rate_to_throttle) -> I/2(STE_rate_to_throttle), Damp/3(STE_rate_to_throttle)
  FMS_Out/1 -> Bus Selector/1, Limit_Select/1(FMS_Out)
  Bus Selector/1 -> I/4(reset)  "<reset>"
  Selector1/1 -> Saturation Dynamic/3
  Selector/1 -> Saturation Dynamic/1

== system Controller/Controller/Attitude_Control/Innerloop_Rate_Control/PI_Control/I_Control ==
  err : Inport
  reset : Inport  Port=2
  Constant : Constant  Value=[0;0;0]  OutDataTypeStr=single
  Discrete-Time Integrator : DiscreteIntegrator  ExternalReset=level  InitialConditionSource=external  SampleTime=-1  LimitOutput=on  UpperSaturationLimit=max_i  LowerSaturationLimit=min_i  ICPrevOutput=DiscIntNeverNeededParam  ICPrevScaledInput=DiscIntNeverNeededParam
  Multiply : Product  OutDataTypeStr=Inherit: Same as first input
  Mux : Mux  Inputs=3
  gain1 : Constant  Value=p_ki  OutDataTypeStr=single
  gain2 : Constant  Value=q_ki  OutDataTypeStr=single
  gain3 : Constant  Value=r_ki  OutDataTypeStr=single
  i_out : Outport  VectorParamsAs1DForOutWhenUnconnected=off
  wires:
  err/1 -> Multiply/2
  gain2/1 -> Mux/2
  gain1/1 -> Mux/1
  gain3/1 -> Mux/3
  reset/1 -> Discrete-Time Integrator/2
  Constant/1 -> Discrete-Time Integrator/3
  Discrete-Time Integrator/1 -> i_out/1
  Mux/1 -> Multiply/1
  Multiply/1 -> Discrete-Time Integrator/1

== system Controller/Controller/Attitude_Control/Innerloop_Rate_Control/PI_Control/P_Control ==
  err : Inport
  Multiply : Product  OutDataTypeStr=Inherit: Same as first input
  Mux : Mux  Inputs=3
  gain1 : Constant  Value=p_kp  OutDataTypeStr=single
  gain2 : Constant  Value=q_kp  OutDataTypeStr=single
  gain3 : Constant  Value=r_kp  OutDataTypeStr=single
  p_out : Outport  VectorParamsAs1DForOutWhenUnconnected=off
  wires:
  err/1 -> Multiply/2
  gain2/1 -> Mux/2
  Mux/1 -> Multiply/1
  gain1/1 -> Mux/1
  Multiply/1 -> p_out/1
  gain3/1 -> Mux/3

== system Controller/Controller/Attitude_Control/Outloop_Angle_Control/Attitude_Controller/Error ==
  att_cmd : Inport
  INS_Out : Inport  Port=2
  Bus_Select : Subsystem
  Demux : Demux  Outputs=2
  Mux : Mux  Inputs=2
  Pitch Offset : Bias  Bias=CONTROL_PARAM.FW_PSP_OFF  SaturateOnIntegerOverflow=off
  Sum : Sum  Inputs=|+-
  euler_err_rad : Outport  VectorParamsAs1DForOutWhenUnconnected=off
  wires:
  att_cmd/1 -> Demux/1  "att_cmd_B_rad"
  Sum/1 -> euler_err_rad/1  "att_error_B_rad"
  INS_Out/1 -> Bus_Select/1(INS_Out)
  Bus_Select/1(att_est_B_rad) -> Sum/2  "att_est_B_rad"
  Demux/2 -> Pitch Offset/1
  Demux/1 -> Mux/1
  Pitch Offset/1 -> Mux/2
  Mux/1 -> Sum/1

== system Controller/Controller/Attitude_Control/Outloop_Angle_Control/Attitude_Controller/P_Controller ==
  error : Inport
  Constant1 : Constant  Value=CONTROL_PARAM.ROLL_P
  Constant2 : Constant  Value=CONTROL_PARAM.PITCH_P
  Multiply : Product
  Mux : Mux  Inputs=2
  u : Outport  VectorParamsAs1DForOutWhenUnconnected=off
  wires:
  Multiply/1 -> u/1
  error/1 -> Multiply/1
  Mux/1 -> Multiply/2
  Constant1/1 -> Mux/1
  Constant2/1 -> Mux/2

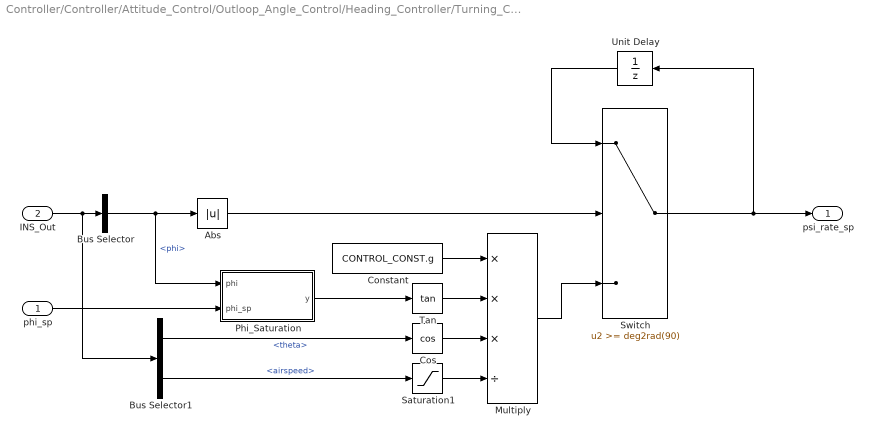
== system Controller/Controller/Attitude_Control/Outloop_Angle_Control/Heading_Controller/Turning_Coordination ==
  phi_sp : Inport
  INS_Out : Inport  Port=2
  Abs : Abs  SaturateOnIntegerOverflow=off
  Bus Selector : BusSelector  OutputSignals=phi
  Bus Selector1 : BusSelector  OutputSignals=theta,airspeed
  Constant : Constant  Value=CONTROL_CONST.g  OutDataTypeStr=single
  Cos : Trigonometry  Operator=cos
  Multiply : Product  Inputs=***/
  Phi_Saturation : Subsystem
  Saturation1 : Saturate  UpperLimit=CONTROL_PARAM.FW_AIRSPD_MAX  LowerLimit=CONTROL_PARAM.FW_AIRSPD_STALL
  Switch : Switch  Threshold=deg2rad(90)  SaturateOnIntegerOverflow=off  InputSameDT=off
  Tan : Trigonometry  Operator=tan
  Unit Delay : UnitDelay  SampleTime=-1  HasFrameUpgradeWarning=on
  psi_rate_sp : Outport  VectorParamsAs1DForOutWhenUnconnected=off
  wires:
  Tan/1 -> Multiply/2
  Cos/1 -> Multiply/3
  Bus Selector/1 -> Phi_Saturation/1(phi), Abs/1  "<phi>"
  INS_Out/1 -> Bus Selector/1, Bus Selector1/1
  Bus Selector1/1 -> Cos/1  "<theta>"
  Abs/1 -> Switch/2
  Unit Delay/1 -> Switch/1
  Multiply/1 -> Switch/3
  Switch/1 -> Unit Delay/1, psi_rate_sp/1
  Constant/1 -> Multiply/1
  Saturation1/1 -> Multiply/4
  Bus Selector1/2 -> Saturation1/1  "<airspeed>"
  phi_sp/1 -> Phi_Saturation/2(phi_sp)
  Phi_Saturation/1(y) -> Tan/1

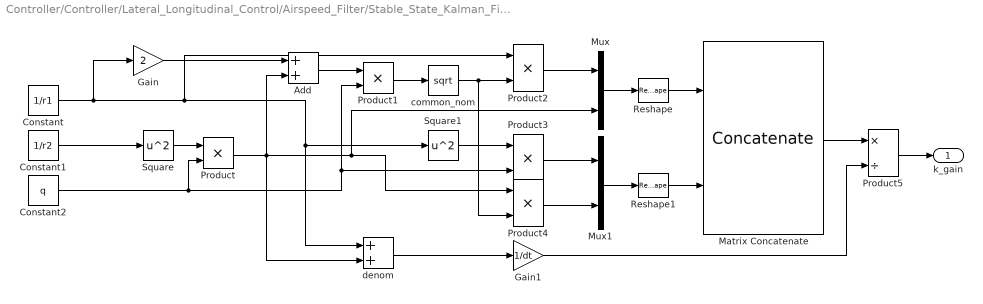
== system Controller/Controller/Lateral_Longitudinal_Control/Airspeed_Filter/Stable_State_Kalman_Filter/Cal_K  ==
  Add : Sum
  Constant : Constant  Value=1/r1  OutDataTypeStr=single
  Constant1 : Constant  Value=1/r2  OutDataTypeStr=single
  Constant2 : Constant  Value=q  OutDataTypeStr=single
  Gain : Gain  Gain=2
  Gain1 : Gain  Gain=1/dt
  Matrix Concatenate : Concatenate  Mode=Multidimensional array
  Mux : Mux  Inputs=2
  Mux1 : Mux  Inputs=2
  Product{,1..4} (5 alike) : Product
  Product5 : Product  Inputs=*/
  Reshape : Reshape  OutputDimensionality=Row vector (2-D)
  Reshape1 : Reshape  OutputDimensionality=Row vector (2-D)
  Square : Math  Operator=square
  Square1 : Math  Operator=square
  common_nom : Sqrt
  denom : Sum
  k_gain : Outport
  wires:
  Constant1/1 -> Square/1
  Square/1 -> Product/1
  Constant2/1 -> Product3/2, Product1/2, Product/2
  Product/1 -> denom/2, Add/2, Product4/1, Mux/2
  Constant/1 -> Gain/1, Product2/1, denom/1, Square1/1
  Gain/1 -> Add/1
  Add/1 -> Product1/1
  Product1/1 -> common_nom/1
  Product2/1 -> Mux/1
  common_nom/1 -> Product4/2, Product2/2
  Mux/1 -> Reshape/1
  Mux1/1 -> Reshape1/1
  Product3/1 -> Mux1/1
  Square1/1 -> Product3/1
  Product4/1 -> Mux1/2
  Matrix Concatenate/1 -> Product5/1
  denom/1 -> Gain1/1
  Product5/1 -> k_gain/1
  Gain1/1 -> Product5/2
  Reshape/1 -> Matrix Concatenate/1
  Reshape1/1 -> Matrix Concatenate/2

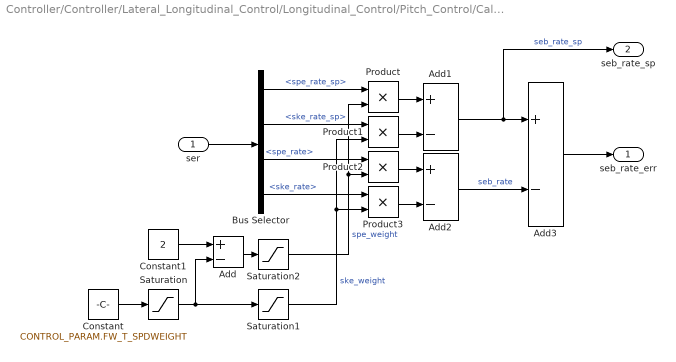
== system Controller/Controller/Lateral_Longitudinal_Control/Longitudinal_Control/Pitch_Control/Calc_Seb_Rate ==
  ser : Inport
  Add{,1..3} (4 alike) : Sum  Inputs=+-
  Bus Selector : BusSelector  OutputSignals=spe_rate_sp,ske_rate_sp,spe_rate,ske_rate
  Constant : Constant  Value=CONTROL_PARAM.FW_T_SPDWEIGHT  OutDataTypeStr=single
  Constant1 : Constant  Value=2  OutDataTypeStr=single
  Product{,1..3} (4 alike) : Product
  Saturation : Saturate  UpperLimit=2  LowerLimit=0
  Saturation1 : Saturate  UpperLimit=1  LowerLimit=0
  Saturation2 : Saturate  UpperLimit=1  LowerLimit=0
  seb_rate_err : Outport
  seb_rate_sp : Outport  Port=2
  wires:
  Saturation2/1 -> Product2/2, Product/2  "spe_weight"
  Add/1 -> Saturation2/1
  Saturation/1 -> Add/2, Saturation1/1
  Saturation1/1 -> Product1/2, Product3/2  "ske_weight"
  Constant1/1 -> Add/1
  Constant/1 -> Saturation/1
  ser/1 -> Bus Selector/1
  Bus Selector/1 -> Product/1  "<spe_rate_sp>"
  Bus Selector/2 -> Product1/1  "<ske_rate_sp>"
  Bus Selector/3 -> Product2/1  "<spe_rate>"
  Bus Selector/4 -> Product3/1  "<ske_rate>"
  Product1/1 -> Add1/2
  Product/1 -> Add1/1
  Product2/1 -> Add2/1
  Product3/1 -> Add2/2
  Add1/1 -> seb_rate_sp/1, Add3/1  "seb_rate_sp"
  Add2/1 -> Add3/2  "seb_rate"
  Add3/1 -> seb_rate_err/1

== system Controller/Controller/Lateral_Longitudinal_Control/Longitudinal_Control/Pitch_Control/FF & Damp ==
  seb_rate_err : Inport
  seb_rate_sp : Inport  Port=2
  Add : Sum
  pitch_damping_gain : Gain  Gain=CONTROL_PARAM.FW_T_PTCH_DAMP
  seb_rate_ff : Gain  Gain=CONTROL_PARAM.FW_T_SEB_R_FF
  ff_d_out : Outport
  wires:
  seb_rate_err/1 -> pitch_damping_gain/1
  seb_rate_sp/1 -> seb_rate_ff/1
  pitch_damping_gain/1 -> Add/1
  seb_rate_ff/1 -> Add/2
  Add/1 -> ff_d_out/1

== system Controller/Controller/Lateral_Longitudinal_Control/Longitudinal_Control/Pitch_Control/I ==
  err : Inport
  maxmin : Inport  Port=2
  reset : Inport  Port=3
  cmd_last : Inport  Port=4
  Discrete-Time Integrator : DiscreteIntegrator  gainval=CONTROL_PARAM.FW_T_I_GAIN_PIT  ExternalReset=level  SampleTime=-1  ICPrevOutput=DiscIntNeverNeededParam  ICPrevScaledInput=DiscIntNeverNeededParam
  Error_Saturation : MATLAB Function  TreatAsAtomicUnit=on
  i_out : Outport
  wires:
  Discrete-Time Integrator/1 -> i_out/1
  maxmin/1 -> Error_Saturation/2(maxmin)
  err/1 -> Error_Saturation/1(err)
  cmd_last/1 -> Error_Saturation/3(cmd_last)
  Error_Saturation/1(res) -> Discrete-Time Integrator/1
  reset/1 -> Discrete-Time Integrator/2

== system Controller/Controller/Lateral_Longitudinal_Control/Longitudinal_Control/Pitch_Control/Limit_Select ==
  FMS_Out : Inport
  Constant : Constant  Value=CONTROL_PARAM.FW_P_LIM_MAX  OutDataTypeStr=single
  Constant1 : Constant  Value=CONTROL_PARAM.FW_P_LIM_MIN  OutDataTypeStr=single
  Mux : Mux  Inputs=2
  Terminator : Terminator
  maxmin : Outport
  wires:
  FMS_Out/1 -> Terminator/1
  Constant/1 -> Mux/1
  Constant1/1 -> Mux/2
  Mux/1 -> maxmin/1

== system Controller/Controller/Lateral_Longitudinal_Control/Longitudinal_Control/Pitch_Control/Pitch_Saturation ==
  note: saturation
  tas : Inport
  ctrl_out : Inport  Port=2
  maxmin : Inport  Port=3
  cmd_last : Inport  Port=4
  Constant : Constant  Value=CONTROL_CONST.g
  Pitch_Saturation : MATLAB Function  TreatAsAtomicUnit=on  mask{dt=CONTROL_CONST.dt, limit=CONTROL_PARAM.FW_T_VERT_ACC}
      mask prompts: limit "vert_accel_limit"
  Product : Product  Inputs=/*
  Saturation Dynamic : simulink/Discontinuities/Saturation Dynamic  OutMin=[]  OutMax=[]  OutDataTypeStr=Inherit: Same as second input  OutDataType=fixdt(1, 16)  OutScaling=2^-10  DoSatur=off
  Selector : Selector  InputPortWidth=2  IndexOptions=Index vector (dialog)  Indices=[1]  OutputSizes=1
  Selector1 : Selector  InputPortWidth=2  IndexOptions=Index vector (dialog)  Indices=[2]  OutputSizes=1
  climb_angle_to_SEB_rate : Product
  tas1 : InportShadow
  pitch_cmd : Outport
  wires:
  climb_angle_to_SEB_rate/1 -> Product/1
  Saturation Dynamic/1 -> Pitch_Saturation/1(u)
  tas/1 -> climb_angle_to_SEB_rate/2
  ctrl_out/1 -> Product/2
  Constant/1 -> climb_angle_to_SEB_rate/1
  Product/1 -> Saturation Dynamic/2
  cmd_last/1 -> Pitch_Saturation/3(y_last)
  Pitch_Saturation/1(y) -> pitch_cmd/1
  tas1/1 -> Pitch_Saturation/2(tas)
  Selector/1 -> Saturation Dynamic/1
  Selector1/1 -> Saturation Dynamic/3
  maxmin/1 -> Selector1/1, Selector/1

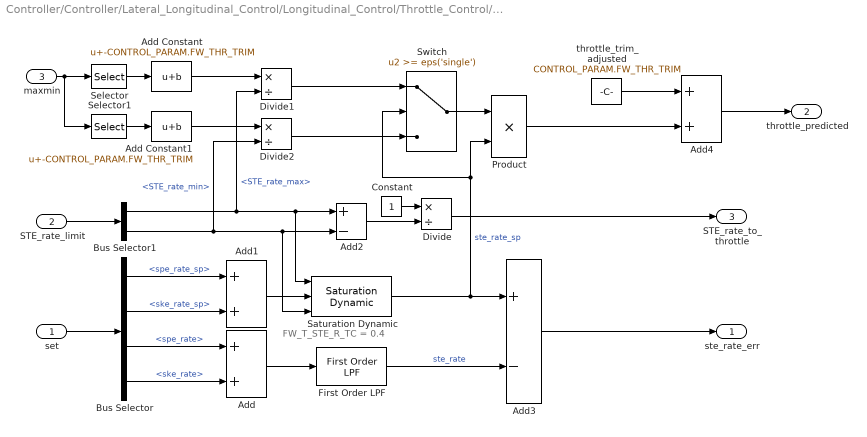
== system Controller/Controller/Lateral_Longitudinal_Control/Longitudinal_Control/Throttle_Control/Calc_STE_Rate ==
  note: FW_T_STE_R_TC = 0.4
  set : Inport
  STE_rate_limit : Inport  Port=2
  maxmin : Inport  Port=3
  Add : Sum
  Add Constant : Bias  Bias=-CONTROL_PARAM.FW_THR_TRIM  SaturateOnIntegerOverflow=off
  Add Constant1 : Bias  Bias=-CONTROL_PARAM.FW_THR_TRIM  SaturateOnIntegerOverflow=off
  Add1 : Sum
  Add2 : Sum  Inputs=+-
  Add3 : Sum  Inputs=+-
  Add4 : Sum
  Bus Selector : BusSelector  OutputSignals=spe_rate_sp,ske_rate_sp,spe_rate,ske_rate
  Bus Selector1 : BusSelector  OutputSignals=STE_rate_max,STE_rate_min
  Constant : Constant  OutDataTypeStr=single
  Divide : Product  Inputs=*/
  Divide1 : Product  Inputs=*/
  Divide2 : Product  Inputs=*/
  First Order LPF : FMT_Model_Lib/Filter/First Order LPF  fc=1/(2*pi*0.4)
      settings: SourceProductName=FMT Toolbox
  Product : Product
  Saturation Dynamic : simulink/Discontinuities/Saturation Dynamic  OutMin=[]  OutMax=[]  OutDataTypeStr=Inherit: Same as second input  OutDataType=fixdt(1, 16)  OutScaling=2^-10  DoSatur=off
  Selector : Selector  InputPortWidth=2  IndexOptions=Index vector (dialog)  Indices=[1]  OutputSizes=1
  Selector1 : Selector  InputPortWidth=2  IndexOptions=Index vector (dialog)  Indices=[2]  OutputSizes=1
  Switch : Switch  Threshold=eps('single')  SaturateOnIntegerOverflow=off  InputSameDT=off
  throttle_trim_adjusted : Constant  Value=CONTROL_PARAM.FW_THR_TRIM  OutDataTypeStr=single
  ste_rate_err : Outport
  throttle_predicted : Outport  Port=2
  STE_rate_to_throttle : Outport  Port=3
  wires:
  Bus Selector1/1 -> Add2/1, Saturation Dynamic/1, Divide1/2  "<STE_rate_max>"
  Bus Selector/3 -> Add/1  "<spe_rate>"
  Add/1 -> First Order LPF/1
  Bus Selector/2 -> Add1/2  "<ske_rate_sp>"
  Add1/1 -> Saturation Dynamic/2
  Bus Selector/4 -> Add/2  "<ske_rate>"
  Bus Selector1/2 -> Add2/2, Saturation Dynamic/3, Divide2/2  "<STE_rate_min>"
  Bus Selector/1 -> Add1/1  "<spe_rate_sp>"
  STE_rate_limit/1 -> Bus Selector1/1
  set/1 -> Bus Selector/1
  First Order LPF/1 -> Add3/2  "ste_rate"
  Saturation Dynamic/1 -> Add3/1, Switch/2, Product/2  "ste_rate_sp"
  Add3/1 -> ste_rate_err/1
  Add2/1 -> Divide/2
  Constant/1 -> Divide/1
  Divide/1 -> STE_rate_to_throttle/1
  Add Constant1/1 -> Divide2/1
  Divide2/1 -> Switch/3
  Divide1/1 -> Switch/1
  Switch/1 -> Product/1
  throttle_trim_adjusted/1 -> Add4/1
  Product/1 -> Add4/2
  Add4/1 -> throttle_predicted/1
  maxmin/1 -> Selector1/1, Selector/1
  Selector/1 -> Add Constant/1
  Add Constant/1 -> Divide1/1
  Selector1/1 -> Add Constant1/1

== system Controller/Controller/Lateral_Longitudinal_Control/Longitudinal_Control/Throttle_Control/Calc_Total_Energy_Rate_Limit ==
  Bus Creator : BusCreator  Inputs=2
  Constant : Constant  Value=CONTROL_CONST.g
  Gain : Gain  Gain=CONTROL_PARAM.FW_T_CLMB_MAX
  Gain1 : Gain  Gain=-CONTROL_PARAM.FW_T_SINK_MIN
  STE_rate_limit : Outport
  wires:
  Constant/1 -> Gain1/1, Gain/1
  Gain/1 -> Bus Creator/1  "STE_rate_max"
  Gain1/1 -> Bus Creator/2  "STE_rate_min"
  Bus Creator/1 -> STE_rate_limit/1

== system Controller/Controller/Lateral_Longitudinal_Control/Longitudinal_Control/Throttle_Control/Damp ==
  ste_rate_err : Inport
  throttle_predicted : Inport  Port=2
  STE_rate_to_throttle : Inport  Port=3
  Add : Sum
  Product : Product
  throttle_damping_gain : Gain  Gain=CONTROL_PARAM.FW_T_THR_DAMP
  ff_d_out : Outport
  wires:
  ste_rate_err/1 -> throttle_damping_gain/1
  throttle_damping_gain/1 -> Product/1
  throttle_predicted/1 -> Add/2
  Add/1 -> ff_d_out/1
  Product/1 -> Add/1
  STE_rate_to_throttle/1 -> Product/2

== system Controller/Controller/Lateral_Longitudinal_Control/Longitudinal_Control/Throttle_Control/I ==
  ste_rate_err : Inport
  STE_rate_to_throttle : Inport  Port=2
  maxmin : Inport  Port=3
  reset : Inport  Port=4
  cmd_last : Inport  Port=5
  Discrete-Time Integrator : DiscreteIntegrator  gainval=CONTROL_PARAM.FW_T_I_GAIN_THR  ExternalReset=level  SampleTime=-1  ICPrevOutput=DiscIntNeverNeededParam  ICPrevScaledInput=DiscIntNeverNeededParam
  Error_Saturation : MATLAB Function  TreatAsAtomicUnit=on
  Product : Product
  i_out : Outport
  wires:
  Discrete-Time Integrator/1 -> i_out/1
  cmd_last/1 -> Error_Saturation/3(cmd_last)
  ste_rate_err/1 -> Product/1
  STE_rate_to_throttle/1 -> Product/2
  maxmin/1 -> Error_Saturation/2(maxmin)
  Error_Saturation/1(res) -> Discrete-Time Integrator/1
  Product/1 -> Error_Saturation/1(err)
  reset/1 -> Discrete-Time Integrator/2

== system Controller/Controller/Lateral_Longitudinal_Control/Longitudinal_Control/Throttle_Control/Limit_Select ==
  FMS_Out : Inport
  Constant : Constant  Value=CONTROL_PARAM.FW_THR_MAX  OutDataTypeStr=single
  Constant1 : Constant  Value=CONTROL_PARAM.FW_THR_MIN  OutDataTypeStr=single
  Mux : Mux  Inputs=2
  Terminator : Terminator
  maxmin : Outport
  wires:
  FMS_Out/1 -> Terminator/1
  Constant/1 -> Mux/1
  Constant1/1 -> Mux/2
  Mux/1 -> maxmin/1

== system Controller/Controller/Attitude_Control/Outloop_Angle_Control/Attitude_Controller/Error/Bus_Select ==
  INS_Out : Inport
  Bus Selector1 : BusSelector  OutputSignals=phi,theta
  Mux1 : Mux  Inputs=2
  att_est_B_rad : Outport  VectorParamsAs1DForOutWhenUnconnected=off
  wires:
  Bus Selector1/2 -> Mux1/2  "<theta>"
  Bus Selector1/1 -> Mux1/1  "<phi>"
  Mux1/1 -> att_est_B_rad/1
  INS_Out/1 -> Bus Selector1/1

== system Controller/Controller/Attitude_Control/Outloop_Angle_Control/Heading_Controller/Turning_Coordination/Phi_Saturation ==
  phi : Inport
  phi_sp : Inport  Port=2
  Abs1 : Abs  SaturateOnIntegerOverflow=off
  Gain : Gain  Gain=-1
  Saturation Dynamic : simulink/Discontinuities/Saturation Dynamic  OutMin=[]  OutMax=[]  OutDataTypeStr=Inherit: Same as second input  OutDataType=fixdt(1, 16)  OutScaling=2^-10  DoSatur=off
  Saturation2 : Saturate  UpperLimit=deg2rad(80)  LowerLimit=-deg2rad(80)
  y : Outport
  wires:
  Gain/1 -> Saturation Dynamic/3
  Abs1/1 -> Gain/1, Saturation Dynamic/1
  phi/1 -> Saturation2/1
  phi_sp/1 -> Abs1/1
  Saturation2/1 -> Saturation Dynamic/2
  Saturation Dynamic/1 -> y/1

== matlab function Controller/Lateral_Longitudinal_Control/Longitudinal_Control/Pitch_Control/Pitch_Saturation/Pitch_Saturation ==
  data: u input; tas input; y output; limit parameter; dt parameter; y_last input
function y = fcn(u, tas, limit, dt, y_last)
pitch_increment = dt * limit / max(tas, eps('single'));
u_min = y_last - pitch_increment;
u_max = y_last + pitch_increment;
if u < u_min
    y = u_min;
else 
    if u > u_max
        y = u_max;
    else
        y = u;
    end
end

== matlab function Controller/Lateral_Longitudinal_Control/Longitudinal_Control/Pitch_Control/I/Error_Saturation ==
  data: err input; res output; maxmin input; cmd_last input
function res = fcn(err, maxmin, cmd_last)

if cmd_last >= maxmin(1)
    err = min(err, 0);
elseif cmd_last <= maxmin(2)
    err = max(err, 0);
end
res = err;

end

== matlab function Controller/Lateral_Longitudinal_Control/Longitudinal_Control/Throttle_Control/I/Error_Saturation ==
  data: err input; res output; maxmin input; cmd_last input
function res = fcn(err, maxmin, cmd_last)

if cmd_last >= maxmin(1)
    err = min(err, 0);
elseif cmd_last <= maxmin(2)
    err = max(err, 0);
end
res = err;

end

== matlab function Controller/Lateral_Longitudinal_Control/Altitude_Control/Calc_Height_Rate_Setpoint/signNoZero ==
  data: u input; y output
function y = fcn(u)

y = single((0) <= u) - (u < (0));
